simulink model "MATE_9LevelDrive_LowHarmonicRectifier"  (R2024b)
settings: Solver=FixedStepDiscrete  StartTime=0.0  StopTime=1  FixedStep=Ts  RelTol=1e-3
PostLoadFcn:
  | Ts=25e-6; initDrive9Level;Rsnu=30; Csnu=3e-6;Ron=0.01;Roff=1e6; Vf=2;
InitFcn:
  | Ts=25e-6; initDrive9Level;Rsnu=30; Csnu=3e-6;Ron=0.01;Roff=1e6; Vf=2;
values from neighbouring files (symbols this model uses):
  Lbase = Zbase/wbase    (= 0.0044902914611)    [initDrive9Level.m]
  Rgnd_rectifier = 1e4    (= 10000)    [initDrive9Level.m]
  T_2wind_ratio = 0.2677    [initDrive9Level.m]
  T_Lpu = Ltot_pu*9/10    (= 0.036)    [initDrive9Level.m]
  T_Lpu_pri = Ltot_pu/10    (= 0.004)    [initDrive9Level.m]
  T_Rpu = Rtot_pu*9/10    (= 0.009)    [initDrive9Level.m]
  T_Rpu_pri = Rtot_pu/10    (= 0.001)    [initDrive9Level.m]
  T_Vpri = 3000    [initDrive9Level.m]
  T_Vpri_15comp = 1.1168    [initDrive9Level.m]
  T_Vsec = 920    [initDrive9Level.m]
  Zbase = T_Vsec*T_Vsec/T_Pbase    (= 1.6928)    [initDrive9Level.m]
undefined symbols (not defined in the file or in its folder): DiscIntNeverNeededParam, gcbh, sps_rtmsupport
libraries: fl_lib x192, ee_lib x105, simetranss x26, nesl_utility x21
(part 1 of 5)
Description:
  | OHV Parallel Inverter Real-Time Simulator
settings Model: ARTEMISmethode_block_infos=$$__separator__$$  Creator=Kyle
settings SolverCC: AlgebraicLoopSolver=TrustRegion
settings DataIOCC: InitialState=xFinal  LimitDataPoints=on  MaxDataPoints=5000  SaveFormat=StructureWithTime  SignalLoggingSaveFormat=ModelDataLogs  SaveOutput=off  SaveTime=off  ReturnWorkspaceOutputs=off  SignalLoggingName=sigsOut
settings OptimizationCC: BlockReduction=off  BooleanDataType=off  OptimizeBlockIOStorage=off  BufferReuse=off  GlobalBufferReuse=off  ExpressionFolding=off  ExpressionDepthLimit=2147483647  LocalBlockOutputs=off  InitFltsAndDblsToZero=on  LifeSpan=inf
settings DebuggingCC: SaveWithParameterizedLinksMsg=none  UnderspecifiedInitializationDetection=Classic  MergeDetectMultiDrivingBlocksExec=none  SignalResolutionControl=TryResolveAllWithWarning  MultiTaskDSMMsg=warning  MultiTaskCondExecSysMsg=none  FcnCallInpInsideContextMsg=warning  UnconnectedInputMsg=warning  UnconnectedOutputMsg=warning  UnconnectedLineMsg=warning  AllowSymbolicDim=off  StateNameClashWarn=warning  SFUnexpectedBacktrackingDiag=warning  SFNoUnconditionalDefaultTransitionDiag=warning  SFExecutionAtInitializationDiag=none  ArithmeticOperatorsInVariantConditions=warning
settings HardwareCC: ProdBitPerPointer=32  ProdBitPerSizeT=32  ProdBitPerPtrDiffT=32  ProdLargestAtomicFloat=None  ProdIntDivRoundTo=Undefined  ProdEndianess=Unspecified  ProdWordSize=32  ProdHWDeviceType=32-bit Generic  TargetUnknown=on
settings ModelReferenceCC: EnableRefExpFcnMdlSchedulingChecks=on  PropagateSignalLabelsOutOfModel=off
settings SFSimCC: SimUseLocalCustomCode=off  CustomCodeUndefinedFunction=UseInterfaceOnly
settings RTWCC: RTWUseLocalCustomCode=off  GPUComputeCapability=3.5
settings CodeAppCC: StateflowObjectComments=on
settings GRTTargetCC: TargetFcnLib=ansi_tfl_tmw.mat  TargetLangStandard=C89/C90 (ANSI)  CombineOutputUpdateFcns=off  GRTInterface=on
settings ConfigComp: CovMetricSettings=dw  CovSaveCumulativeToWorkspaceVar=on  CovSaveSingleToWorkspaceVar=on  CovExternalEMLEnable=off
settings SimscapeCC: SimscapeNormalizeSystem=off

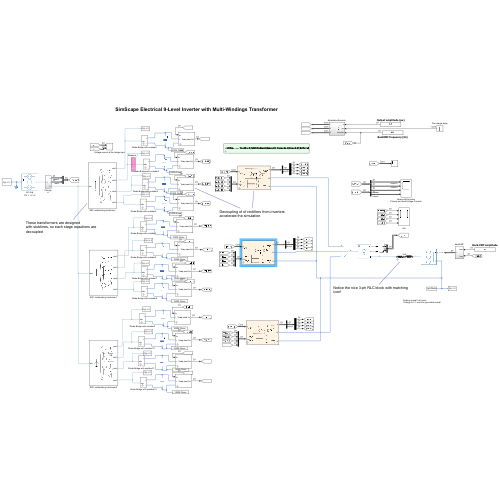
[thumbnail: Simulink's stored preview of the top-level diagram]
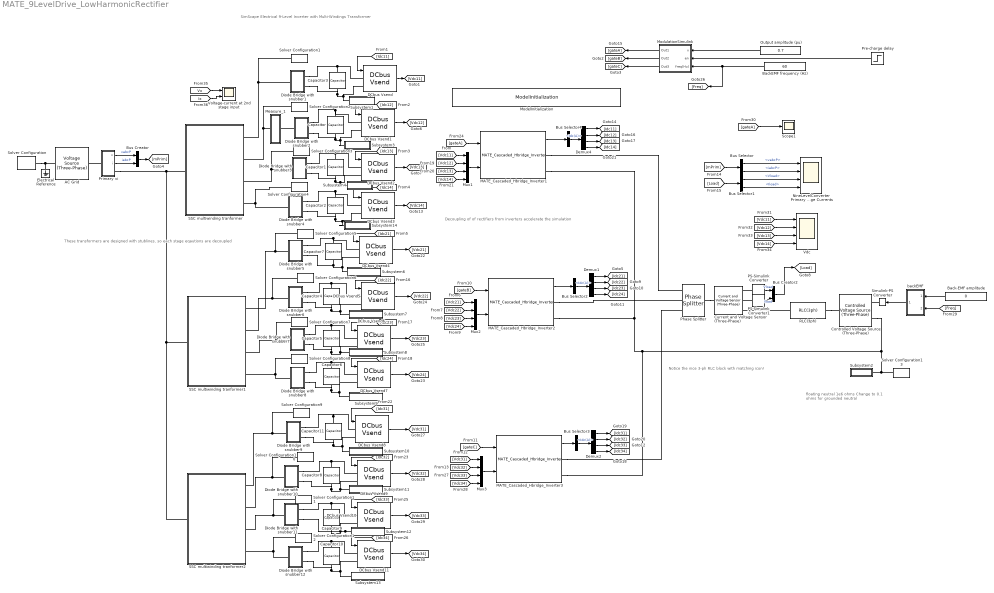
== system MATE_9LevelDrive_LowHarmonicRectifier ==
  note: Decoupling of of rectifiers from inverters
      | accelerate the simulation
  note: floating neutral 1e6 ohms
      | Change to 0.1 ohms for grounded neutral
  note: SimScape Electrical 9-Level Inverter with Multi-Windings Transformer
  note: These transformers are designed
      | with stublines, so each stage eqautions are decoupled
  note: Notice the nice 3-ph RLC block with matching icon!
  AC Grid : ee_lib/Sources/Voltage Source (Three-Phase)  vline_rms=120*sqrt(3) V  shift=0 deg  freq=60 Hz  impedance_option=1  SShortCircuit=1e6 A*V  XR=15  R=0.01 Ohm  L=3.97e-4 H  harmonic_option=0  harmonic_orders=[5.0, 7.0, 11.0, 13.0]  harmonic_ratios=[0.1, 0.1, 0.1, 0.1]  G_parasitic=0 1/Ohm  I_specify=off  I_priority=None  I=[0, 0, 0] A  I_nominal_specify=off  I_nominal_value=1  I_nominal_unit=A
      settings: AttributesFormatString="208 V  60 Hz"
  Back-EMF amplitude : Constant  Value=0
  BackEMF frequency (Hz) : Constant  Value=60
  Bus Creator : BusCreator  Inputs=2
  Bus Creator2 : BusCreator  Inputs=2
  Bus Selector : BusSelector  OutputSignals=vabcP,iabcP
  Bus Selector1 : BusSelector  OutputSignals=Vload,Iload
  Bus Selector2 : BusSelector  OutputSignals=Idc(A)
  Bus Selector3 : BusSelector  OutputSignals=Idc(A)
  Bus Selector4 : BusSelector  OutputSignals=Idc(A)
  Capacitor{,1..11} (12 alike) : fl_lib/Electrical/Electrical Elements/Capacitor  c=Cdclink F  r=Rdclink_series Ohm  g=0 1/Ohm  i_specify=off  i_priority=None  i=0 A  i_nominal_specify=off  i_nominal_value=1  i_nominal_unit=A  v_specify=off  v_priority=None  v=0 V  v_nominal_specify=off  v_nominal_value=1  v_nominal_unit=V  vc_specify=off  vc_priority=High  vc=0 V  vc_nominal_specify=off  vc_nominal_value=1  vc_nominal_unit=V
  Controlled Voltage Source (Three-Phase) : ee_lib/Sources/Controlled Voltage Source (Three-Phase)  input_option=ee.enum.inputType.instantaneous  FRated=60 Hz
      settings: InternalSimscapePortConfiguration="{\"Bottom\":[],\"Left\":[{\"id\":\"S\",\"label\":\"S\",\"type\":\"input\"},{\"id\":\"n\",\"label\":\"n\",\"type\":\"foundation.electrical.electrical\"}],\"Right\":[{\"id\":\"N\",\"label\":\"~\",\"type\":\"foundation.electrical.three_phase\"}],\"Top\":[]}"
  Current and Voltage Sensor (Three-Phase) : ee_lib/Sensors & Transducers/Current and Voltage Sensor (Three-Phase)  vMeasurementType=ee.enum.vmeasurement.lg  outputUnit=ee.enum.unit.si  SRated=100e6 A*V  VRated=24e3 V  I_specify=off  I_priority=None  I=[0, 0, 0] A  I_nominal_specify=off  I_nominal_value=1  I_nominal_unit=A  V_specify=off  V_priority=None  V=[0, 0, 0] V  V_nominal_specify=off  V_nominal_value=1  V_nominal_unit=V
      settings: InternalSimscapePortConfiguration="{\"Bottom\":[],\"Left\":[{\"id\":\"N1\",\"label\":\"~1\",\"type\":\"foundation.electrical.three_phase\"}],\"Right\":[{\"id\":\"V_output\",\"label\":\"V\",\"type\":\"output\"},{\"id\":\"I_output\",\"label\":\"I\",\"type\":\"output\"},{\"id\":\"N2\",\"label\":\"~2\",\"type\":\"foundation.electrical.three_phase\"}],\"Top\":[]}"
  DCbus Vsend{,1..11} (12 alike) : simetranss/Network decoupling/DCbus Vsend  Ts=Ts
  Demux1 : Demux
      settings: DisplayOption=none
  Demux2 : Demux
      settings: DisplayOption=none
  Demux4 : Demux
      settings: DisplayOption=none
  Diode Bridge with snubber1 : Subsystem  mask(MATE 3-phase Diode/Thyristor Rectifier){rsnu=Rsnu, csnu=Csnu}
      mask prompts: rsnu "Snubber resistance (Ohms)"; csnu "Snubber capacitance (Ohms)"
  Diode Bridge with snubber10 : Subsystem  mask(MATE 3-phase Diode/Thyristor Rectifier){rsnu=Rsnu, csnu=Csnu}
      mask prompts: rsnu "Snubber resistance (Ohms)"; csnu "Snubber capacitance (Ohms)"
  Diode Bridge with snubber11 : Subsystem  mask(MATE 3-phase Diode/Thyristor Rectifier){rsnu=Rsnu, csnu=Csnu}
      mask prompts: rsnu "Snubber resistance (Ohms)"; csnu "Snubber capacitance (Ohms)"
  Diode Bridge with snubber12 : Subsystem  mask(MATE 3-phase Diode/Thyristor Rectifier){rsnu=Rsnu, csnu=Csnu}
      mask prompts: rsnu "Snubber resistance (Ohms)"; csnu "Snubber capacitance (Ohms)"
  Diode Bridge with snubber2 : Subsystem  mask(MATE 3-phase Diode/Thyristor Rectifier){rsnu=Rsnu, csnu=Csnu}
      mask prompts: rsnu "Snubber resistance (Ohms)"; csnu "Snubber capacitance (Ohms)"
  Diode Bridge with snubber3 : Subsystem  mask(MATE 3-phase Diode/Thyristor Rectifier){rsnu=Rsnu, csnu=Csnu}
      mask prompts: rsnu "Snubber resistance (Ohms)"; csnu "Snubber capacitance (Ohms)"
  Diode Bridge with snubber4 : Subsystem  mask(MATE 3-phase Diode/Thyristor Rectifier){rsnu=Rsnu, csnu=Csnu}
      mask prompts: rsnu "Snubber resistance (Ohms)"; csnu "Snubber capacitance (Ohms)"
  Diode Bridge with snubber5 : Subsystem  mask(MATE 3-phase Diode/Thyristor Rectifier){rsnu=Rsnu, csnu=Csnu}
      mask prompts: rsnu "Snubber resistance (Ohms)"; csnu "Snubber capacitance (Ohms)"
  Diode Bridge with snubber6 : Subsystem  mask(MATE 3-phase Diode/Thyristor Rectifier){rsnu=Rsnu, csnu=Csnu}
      mask prompts: rsnu "Snubber resistance (Ohms)"; csnu "Snubber capacitance (Ohms)"
  Diode Bridge with snubber7 : Subsystem  mask(MATE 3-phase Diode/Thyristor Rectifier){rsnu=Rsnu, csnu=Csnu}
      mask prompts: rsnu "Snubber resistance (Ohms)"; csnu "Snubber capacitance (Ohms)"
  Diode Bridge with snubber8 : Subsystem  mask(MATE 3-phase Diode/Thyristor Rectifier){rsnu=Rsnu, csnu=Csnu}
      mask prompts: rsnu "Snubber resistance (Ohms)"; csnu "Snubber capacitance (Ohms)"
  Diode Bridge with snubber9 : Subsystem  mask(MATE 3-phase Diode/Thyristor Rectifier){rsnu=Rsnu, csnu=Csnu}
      mask prompts: rsnu "Snubber resistance (Ohms)"; csnu "Snubber capacitance (Ohms)"
  Electrical Reference : fl_lib/Electrical/Electrical Elements/Electrical Reference
  MATE_Cascaded_Hbridge_Inverter1 : simetranss/Power converters/MATE_Cascaded_Hbridge_Inverter  Gtype=Mean Active Duty (0<=g<=1)  nbc=4  ron=0.001  roff=1e5  Ts=Ts
  MATE_Cascaded_Hbridge_Inverter2 : simetranss/Power converters/MATE_Cascaded_Hbridge_Inverter  Gtype=Mean Active Duty (0<=g<=1)  nbc=4  ron=0.001  roff=1e5  Ts=Ts
  MATE_Cascaded_Hbridge_Inverter3 : simetranss/Power converters/MATE_Cascaded_Hbridge_Inverter  Gtype=Mean Active Duty (0<=g<=1)  nbc=4  ron=0.001  roff=1e5  Ts=Ts
  Measure_1 : Subsystem  DialogController=POWERSYS.PowerSysDialog  StartFcn=sps_rtmsupport('StartFcn',gcbh);  StopFcn=sps_rtmsupport('StopFcn',gcbh);  mask(Three-Phase Measurement){Va=Vx, Ia=Ix}
      mask prompts: Va "Voltage signal label  (use a From block to collect this signal)"; Ia "Current signal label  (use a From block to collect this signal)"
      mask help:
      | Ideal three-phase voltage and current measurements.
      |
      | The block outputs the voltages and currents in volts and amperes at the corresponding From blocks
      mask init:
      | bloc = gcb;
      | 
      | Vtag=get_param(bloc,'Va');
      | Itag=get_param(bloc,'Ia');
      | 
      | set_param([bloc '/Vabc'],'GotoTag',[Vtag]);
      | set_param([bloc '/Iabc'],'GotoTag',[Itag]);
      settings: UndoDeleteFcn=sps_rtmsupport('UndoDeleteFcn',gcbh);
      mask Help: helpview(psbhelp)
  ModelInitialization : simetranss/Usefulls/ModelInitialization  InitFcnX=Ts=25e-6; initDrive9Level;Rsnu=30; Csnu=3e-6;Ron=0.01;Roff=1e6; Vf=2;  prel=off  posl=on  inif=on  strf=off
  ModulationSimulink : Subsystem
  Mux1 : Mux
  Mux2 : Mux
  Mux3 : Mux
  NineLevelConverter Primary and load Voltage Currents : Scope  NumInputPorts=4
  Output amplitude (pu) : Constant  Value=0.7
  PS-Simulink Converter : nesl_utility/PS-Simulink Converter  PhysicalDomain=network_engine_domain  SubClassName=ps_output  LeftPortType=input  RightPortType=output  PseudoPeriodic=off  Frequencies=[]  VectorFormat=1-D array  Unit=V  AffineConversion=off
  PS-Simulink Converter1 : nesl_utility/PS-Simulink Converter  PhysicalDomain=network_engine_domain  SubClassName=ps_output  LeftPortType=input  RightPortType=output  PseudoPeriodic=off  Frequencies=[]  VectorFormat=1-D array  Unit=A  AffineConversion=off
  Phase Splitter : ee_lib/Connectors & References/Phase Splitter
  Pre-charge delay : Step  Time=0.2  SampleTime=0
  Primary vi : Subsystem
  RLC(3ph) : simetranss/Passive/RLC(3ph)  BranchType=RL  SerPar=Series  Resistance=5  Inductance=6e-3  Capacitance=1e-6  Ropen=1e9
  SSC multiwinding tranformer : Subsystem
  SSC multiwinding tranformer1 : Subsystem
  SSC multiwinding tranformer2 : Subsystem
  Scope1 : Scope
  Simulink-PS Converter : nesl_utility/Simulink-PS Converter  PhysicalDomain=network_engine_domain  SubClassName=ps_input  LeftPortType=input  RightPortType=output  PseudoPeriodic=off  Frequencies=[]  NoiseDistribution=none  NoiseParameters=[]  Unit=1  AffineConversion=off  FilteringAndDerivatives=provide  SimscapeFilterOrder=1  InputFilterTimeConstant=0.001  UdotUserProvided=0
  Solver Configuration : nesl_utility/Solver Configuration  PhysicalDomain=network_engine_domain  SubClassName=solver  LeftPortType=input  RightPortType=generic  Tones=[]  Harmonics=[]  SimulateNoise=off  Profile=off  UseLocalSampling=off  EnableSwitchedLinearOptims=on  FrequencyDomain=off  UseCCode=off  RelTol=0.001  AbsTol=1e-06  MinStep=1e-09  ToWorkspace=off  RevertToSquareIcSolve=off  NumHomotopyIterations=100  PhasorMode=off  PhasorModeNumHarmonics=1  ConsistencySolver=NEWTON_FTOL  IndexReductionMethod=None  DoDC=off  ResidualTolerance=1e-03  ConsistencyTolSource=GLOBAL  ConsistencyAbsTol=0.001  ConsistencyRelTol=0.001  ConsistencyTolFactor=0.001  UseLocalSolver=on  LocalSolverChoice=NE_BACKWARD_EULER_ADVANCER  ResolveIndetEquations=off  FunctionEvalNumThread=1  LocalSolverSampleTime=Ts  DoFixedCost=on  MaxNonlinIter=1  MaxModeIter=2  ComputeImpulses=off  ImpulseIterations=2  LinearAlgebra=auto  LinearAlgebraNumThread=0  EquationFormulation=NE_TIME_EF  DelaysMemoryBudget=1024  AutomaticFiltering=off  FilteringTimeConstant=0.001  PartitionStorageMethod=AS_NEEDED  PartitionMemoryBudget=1024  PartitionMethod=ROBUST  MultibodyUseLocalSolver=off  MultibodyLocalSolverChoice=ODE1  MultibodyLocalSolverSampleTime=0.001
  Solver Configuration{1..12} (12 alike) : nesl_utility/Solver Configuration  PhysicalDomain=network_engine_domain  SubClassName=solver  LeftPortType=input  RightPortType=generic  Tones=[]  Harmonics=[]  SimulateNoise=off  Profile=off  UseLocalSampling=off  EnableSwitchedLinearOptims=on  FrequencyDomain=off  UseCCode=off  RelTol=0.001  AbsTol=1e-06  MinStep=1e-09  ToWorkspace=off  RevertToSquareIcSolve=off  NumHomotopyIterations=100  PhasorMode=off  PhasorModeNumHarmonics=1  ConsistencySolver=NEWTON_FTOL  IndexReductionMethod=None  DoDC=off  ResidualTolerance=1e-09  ConsistencyTolSource=GLOBAL  ConsistencyAbsTol=0.001  ConsistencyRelTol=0.001  ConsistencyTolFactor=0.001  UseLocalSolver=on  LocalSolverChoice=NE_BACKWARD_EULER_ADVANCER  ResolveIndetEquations=off  FunctionEvalNumThread=1  LocalSolverSampleTime=Ts  DoFixedCost=on  MaxNonlinIter=1  MaxModeIter=2  ComputeImpulses=off  ImpulseIterations=2  LinearAlgebra=auto  LinearAlgebraNumThread=0  EquationFormulation=NE_TIME_EF  DelaysMemoryBudget=1024  AutomaticFiltering=off  FilteringTimeConstant=0.001  PartitionStorageMethod=AS_NEEDED  PartitionMemoryBudget=1024  PartitionMethod=ROBUST  MultibodyUseLocalSolver=off  MultibodyLocalSolverChoice=ODE1  MultibodyLocalSolverSampleTime=0.001
  Solver Configuration13 : nesl_utility/Solver Configuration  PhysicalDomain=network_engine_domain  SubClassName=solver  LeftPortType=input  RightPortType=generic  Tones=[]  Harmonics=[]  SimulateNoise=off  Profile=off  UseLocalSampling=off  EnableSwitchedLinearOptims=on  FrequencyDomain=off  UseCCode=off  RelTol=0.001  AbsTol=1e-06  MinStep=1e-09  ToWorkspace=off  RevertToSquareIcSolve=off  NumHomotopyIterations=100  PhasorMode=off  PhasorModeNumHarmonics=1  ConsistencySolver=NEWTON_FTOL  IndexReductionMethod=None  DoDC=off  ResidualTolerance=1e-03  ConsistencyTolSource=GLOBAL  ConsistencyAbsTol=0.001  ConsistencyRelTol=0.001  ConsistencyTolFactor=0.001  UseLocalSolver=on  LocalSolverChoice=NE_BACKWARD_EULER_ADVANCER  ResolveIndetEquations=off  FunctionEvalNumThread=1  LocalSolverSampleTime=Ts  DoFixedCost=on  MaxNonlinIter=1  MaxModeIter=2  ComputeImpulses=off  ImpulseIterations=2  LinearAlgebra=auto  LinearAlgebraNumThread=0  EquationFormulation=NE_TIME_EF  DelaysMemoryBudget=1024  AutomaticFiltering=off  FilteringTimeConstant=0.001  PartitionStorageMethod=AS_NEEDED  PartitionMemoryBudget=1024  PartitionMethod=ROBUST  MultibodyUseLocalSolver=off  MultibodyLocalSolverChoice=ODE1  MultibodyLocalSolverSampleTime=0.001
  Subsystem1 : Subsystem  mask(Ground Referencing Resistor){Rr=Rgnd_rectifier}
      mask prompts: Rr "Resistance (Ohms)"
      mask help: This block is a simple resistance to provide a reference to the ground for the SimScape solver.
      mask init:
      | r=get_param(gcb,'Rr');
      | rr=num2str(Rr);
      | txt=[rr ' Ohms'];
      mask Display: disp(txt)
  Subsystem10 : Subsystem  mask(Ground Referencing Resistor){Rr=Rgnd_rectifier}
      mask prompts: Rr "Resistance (Ohms)"
      mask help: This block is a simple resistance to provide a reference to the ground for the SimScape solver.
      mask init:
      | r=get_param(gcb,'Rr');
      | rr=num2str(Rr);
      | txt=[rr ' Ohms'];
      mask Display: disp(txt)
  Subsystem11 : Subsystem  mask(Ground Referencing Resistor){Rr=Rgnd_rectifier}
      mask prompts: Rr "Resistance (Ohms)"
      mask help: This block is a simple resistance to provide a reference to the ground for the SimScape solver.
      mask init:
      | r=get_param(gcb,'Rr');
      | rr=num2str(Rr);
      | txt=[rr ' Ohms'];
      mask Display: disp(txt)
  Subsystem12 : Subsystem  mask(Ground Referencing Resistor){Rr=Rgnd_rectifier}
      mask prompts: Rr "Resistance (Ohms)"
      mask help: This block is a simple resistance to provide a reference to the ground for the SimScape solver.
      mask init:
      | r=get_param(gcb,'Rr');
      | rr=num2str(Rr);
      | txt=[rr ' Ohms'];
      mask Display: disp(txt)
  Subsystem13 : Subsystem  mask(Ground Referencing Resistor){Rr=Rgnd_rectifier}
      mask prompts: Rr "Resistance (Ohms)"
      mask help: This block is a simple resistance to provide a reference to the ground for the SimScape solver.
      mask init:
      | r=get_param(gcb,'Rr');
      | rr=num2str(Rr);
      | txt=[rr ' Ohms'];
      mask Display: disp(txt)
  Subsystem14 : Subsystem  mask(Ground Referencing Resistor){Rr=Rgnd_rectifier}
      mask prompts: Rr "Resistance (Ohms)"
      mask help: This block is a simple resistance to provide a reference to the ground for the SimScape solver.
      mask init:
      | r=get_param(gcb,'Rr');
      | rr=num2str(Rr);
      | txt=[rr ' Ohms'];
      mask Display: disp(txt)
  Subsystem2 : Subsystem  mask(Ground Referencing Resistor){Rr=1e6}
      mask prompts: Rr "Resistance (Ohms)"
      mask help: This block is a simple resistance to provide a reference to the ground for the SimScape solver.
      mask init:
      | r=get_param(gcb,'Rr');
      | txt=[r ' Ohms'];
      mask Display: disp(txt)
  Subsystem3 : Subsystem  mask(Ground Referencing Resistor){Rr=Rgnd_rectifier}
      mask prompts: Rr "Resistance (Ohms)"
      mask help: This block is a simple resistance to provide a reference to the ground for the SimScape solver.
      mask init:
      | r=get_param(gcb,'Rr');
      | rr=num2str(Rr);
      | txt=[rr ' Ohms'];
      mask Display: disp(txt)
  Subsystem4 : Subsystem  mask(Ground Referencing Resistor){Rr=Rgnd_rectifier}
      mask prompts: Rr "Resistance (Ohms)"
      mask help: This block is a simple resistance to provide a reference to the ground for the SimScape solver.
      mask init:
      | r=get_param(gcb,'Rr');
      | rr=num2str(Rr);
      | txt=[rr ' Ohms'];
      mask Display: disp(txt)
  Subsystem6 : Subsystem  mask(Ground Referencing Resistor){Rr=Rgnd_rectifier}
      mask prompts: Rr "Resistance (Ohms)"
      mask help: This block is a simple resistance to provide a reference to the ground for the SimScape solver.
      mask init:
      | r=get_param(gcb,'Rr');
      | rr=num2str(Rr);
      | txt=[rr ' Ohms'];
      mask Display: disp(txt)
  Subsystem7 : Subsystem  mask(Ground Referencing Resistor){Rr=Rgnd_rectifier}
      mask prompts: Rr "Resistance (Ohms)"
      mask help: This block is a simple resistance to provide a reference to the ground for the SimScape solver.
      mask init:
      | r=get_param(gcb,'Rr');
      | rr=num2str(Rr);
      | txt=[rr ' Ohms'];
      mask Display: disp(txt)
  Subsystem8 : Subsystem  mask(Ground Referencing Resistor){Rr=Rgnd_rectifier}
      mask prompts: Rr "Resistance (Ohms)"
      mask help: This block is a simple resistance to provide a reference to the ground for the SimScape solver.
      mask init:
      | r=get_param(gcb,'Rr');
      | rr=num2str(Rr);
      | txt=[rr ' Ohms'];
      mask Display: disp(txt)
  Subsystem9 : Subsystem  mask(Ground Referencing Resistor){Rr=Rgnd_rectifier}
      mask prompts: Rr "Resistance (Ohms)"
      mask help: This block is a simple resistance to provide a reference to the ground for the SimScape solver.
      mask init:
      | r=get_param(gcb,'Rr');
      | rr=num2str(Rr);
      | txt=[rr ' Ohms'];
      mask Display: disp(txt)
  Vdc : Scope  NumInputPorts=4
  Voltage-current at 2nd stage input : Scope  NumInputPorts=2
  backEMF : Subsystem
  wires:
  Bus Creator/1 -> [mPrim]
  Primary vi/1(v) -> Bus Creator/1  "vabcP"
  Primary vi/2(i) -> Bus Creator/2  "iabcP"
  DCbus Vsend1/1 -> [Vdc12]
  DCbus Vsend2/1 -> [Vdc13]
  DCbus Vsend3/1 -> [Vdc14]
  DCbus Vsend/1 -> [Vdc11]
  Back-EMF amplitude/1 -> backEMF/1(amp)
  backEMF/1(Out1) -> Simulink-PS Converter/1
  BackEMF frequency (Hz)/1 -> [Freq], ModulationSimulink/3(freq(Hz))
  Output amplitude (pu)/1 -> ModulationSimulink/1(x)
  [mPrim] -> Bus Selector/1
  PS-Simulink Converter1/1 -> Bus Creator2/2  "Iload"
  PS-Simulink Converter/1 -> Bus Creator2/1  "Vload"
  Bus Creator2/1 -> [Load]
  [Load] -> Bus Selector1/1
  Bus Selector/2 -> NineLevelConverter Primary and load Voltage Currents/2  "<iabcP>"
  Bus Selector/1 -> NineLevelConverter Primary and load Voltage Currents/1  "<vabcP>"
  Bus Selector1/2 -> NineLevelConverter Primary and load Voltage Currents/4  "<Iload>"
  Bus Selector1/1 -> NineLevelConverter Primary and load Voltage Currents/3  "<Vload>"
  ModulationSimulink/1(Out1) -> [gateA]
  [Vdc11] -> Mux1/1
  [Vdc12] -> Mux1/2
  [Vdc13] -> Mux1/3
  [Vdc14] -> Mux1/4
  Mux1/1 -> MATE_Cascaded_Hbridge_Inverter1/2
  [gateA] -> MATE_Cascaded_Hbridge_Inverter1/1
  MATE_Cascaded_Hbridge_Inverter1/1 -> Bus Selector4/1
  Bus Selector4/1 -> Demux4/1  "<Idc(A)>"
  Demux4/1 -> [Idc11]
  Demux4/2 -> [Idc12]
  Demux4/3 -> [Idc13]
  Demux4/4 -> [Idc14]
  [Idc11] -> DCbus Vsend/1
  [Idc12] -> DCbus Vsend1/1
  [Idc13] -> DCbus Vsend2/1
  [Idc14] -> DCbus Vsend3/1
  Pre-charge delay/1 -> ModulationSimulink/2(en)
  DCbus Vsend4/1 -> [Vdc21]
  DCbus Vsend5/1 -> [Vdc22]
  DCbus Vsend6/1 -> [Vdc23]
  DCbus Vsend7/1 -> [Vdc24]
  [Idc21] -> DCbus Vsend4/1
  [Idc22] -> DCbus Vsend5/1
  [Idc23] -> DCbus Vsend6/1
  [Idc24] -> DCbus Vsend7/1
  DCbus Vsend8/1 -> [Vdc31]
  DCbus Vsend9/1 -> [Vdc32]
  DCbus Vsend10/1 -> [Vdc33]
  DCbus Vsend11/1 -> [Vdc34]
  [Idc31] -> DCbus Vsend8/1
  [Idc32] -> DCbus Vsend9/1
  [Idc33] -> DCbus Vsend10/1
  [Idc34] -> DCbus Vsend11/1
  ModulationSimulink/2(Out2) -> [gateB]
  ModulationSimulink/3(Out3) -> [gateC]
  Demux1/4 -> [Idc24]
  Demux1/3 -> [Idc23]
  Demux1/2 -> [Idc22]
  Demux1/1 -> [Idc21]
  Bus Selector2/1 -> Demux1/1  "<Idc(A)>"
  MATE_Cascaded_Hbridge_Inverter2/1 -> Bus Selector2/1
  [gateB] -> MATE_Cascaded_Hbridge_Inverter2/1
  Mux2/1 -> MATE_Cascaded_Hbridge_Inverter2/2
  [Vdc24] -> Mux2/4
  [Vdc23] -> Mux2/3
  [Vdc22] -> Mux2/2
  [Vdc21] -> Mux2/1
  [Vdc31] -> Mux3/1
  [Vdc32] -> Mux3/2
  [Vdc33] -> Mux3/3
  [Vdc34] -> Mux3/4
  Mux3/1 -> MATE_Cascaded_Hbridge_Inverter3/2
  [gateC] -> MATE_Cascaded_Hbridge_Inverter3/1
  MATE_Cascaded_Hbridge_Inverter3/1 -> Bus Selector3/1
  Bus Selector3/1 -> Demux2/1  "<Idc(A)>"
  Demux2/1 -> [Idc31]
  Demux2/2 -> [Idc32]
  Demux2/3 -> [Idc33]
  Demux2/4 -> [Idc34]
  [Freq] -> backEMF/2(freq)
  [gateA] -> Scope1/1
  [Vdc11] -> Vdc/1
  [Vdc12] -> Vdc/2
  [Vdc13] -> Vdc/3
  [Vdc14] -> Vdc/4
  [Vx] -> Voltage-current at 2nd stage input/1
  [Ix] -> Voltage-current at 2nd stage input/2
  connections:
  AC Grid/LConn1 -- Solver Configuration/RConn1 -- Electrical Reference/LConn1
  Primary vi/RConn1 -- SSC multiwinding tranformer/LConn1 -- SSC multiwinding tranformer2/LConn1 -- SSC multiwinding tranformer1/LConn1
  Primary vi/LConn1 -- AC Grid/RConn1
  Capacitor/LConn1 -- Diode Bridge with snubber2/RConn1 -- DCbus Vsend1/LConn1
  Capacitor/RConn1 -- Diode Bridge with snubber2/RConn2 -- DCbus Vsend1/LConn2 -- Subsystem3/RConn1
  Diode Bridge with snubber3/RConn1 -- DCbus Vsend2/LConn1 -- Capacitor1/LConn1
  Capacitor1/RConn1 -- Diode Bridge with snubber3/RConn2 -- DCbus Vsend2/LConn2 -- Subsystem4/RConn1
  Capacitor2/LConn1 -- DCbus Vsend3/LConn1 -- Diode Bridge with snubber4/RConn1
  Capacitor2/RConn1 -- Diode Bridge with snubber4/RConn2 -- DCbus Vsend3/LConn2 -- Subsystem14/RConn1
  Capacitor3/LConn1 -- DCbus Vsend/LConn1 -- Diode Bridge with snubber1/RConn1
  Capacitor3/RConn1 -- Diode Bridge with snubber1/RConn2 -- DCbus Vsend/LConn2 -- Subsystem1/RConn1
  Diode Bridge with snubber1/LConn1 -- SSC multiwinding tranformer/RConn1 -- Solver Configuration1/RConn1
  Measure_1/LConn1 -- Solver Configuration2/RConn1 -- SSC multiwinding tranformer/RConn2
  Diode Bridge with snubber3/LConn1 -- SSC multiwinding tranformer/RConn3 -- Solver Configuration3/RConn1
  Diode Bridge with snubber4/LConn1 -- Solver Configuration4/RConn1 -- SSC multiwinding tranformer/RConn4
  RLC(3ph)/RConn1 -- Controlled Voltage Source (Three-Phase)/RConn1
  Simulink-PS Converter/RConn1 -- Controlled Voltage Source (Three-Phase)/LConn1
  Phase Splitter/LConn1 -- Current and Voltage Sensor (Three-Phase)/LConn1
  RLC(3ph)/LConn1 -- Current and Voltage Sensor (Three-Phase)/RConn3
  PS-Simulink Converter/LConn1 -- Current and Voltage Sensor (Three-Phase)/RConn1
  PS-Simulink Converter1/LConn1 -- Current and Voltage Sensor (Three-Phase)/RConn2
  Controlled Voltage Source (Three-Phase)/LConn2 -- Solver Configuration13/RConn1 -- Subsystem2/RConn1 -- MATE_Cascaded_Hbridge_Inverter3/RConn2 -- MATE_Cascaded_Hbridge_Inverter2/RConn2 -- MATE_Cascaded_Hbridge_Inverter1/RConn2
  Diode Bridge with snubber6/RConn1 -- DCbus Vsend5/LConn1 -- Capacitor4/LConn1
  Capacitor4/RConn1 -- Diode Bridge with snubber6/RConn2 -- DCbus Vsend5/LConn2 -- Subsystem7/RConn1
  Diode Bridge with snubber7/RConn1 -- DCbus Vsend6/LConn1 -- Capacitor5/LConn1
  Capacitor5/RConn1 -- Diode Bridge with snubber7/RConn2 -- DCbus Vsend6/LConn2 -- Subsystem8/RConn1
  Capacitor6/LConn1 -- DCbus Vsend7/LConn1 -- Diode Bridge with snubber8/RConn1
  Capacitor6/RConn1 -- Diode Bridge with snubber8/RConn2 -- DCbus Vsend7/LConn2 -- Subsystem9/RConn1
  Diode Bridge with snubber5/RConn1 -- DCbus Vsend4/LConn1 -- Capacitor7/LConn1
  Capacitor7/RConn1 -- Diode Bridge with snubber5/RConn2 -- DCbus Vsend4/LConn2 -- Subsystem6/RConn1
  Diode Bridge with snubber8/LConn1 -- Solver Configuration8/RConn1 -- SSC multiwinding tranformer1/RConn4
  Diode Bridge with snubber7/LConn1 -- SSC multiwinding tranformer1/RConn3 -- Solver Configuration7/RConn1
  Diode Bridge with snubber6/LConn1 -- SSC multiwinding tranformer1/RConn2 -- Solver Configuration6/RConn1
  Diode Bridge with snubber5/LConn1 -- SSC multiwinding tranformer1/RConn1 -- Solver Configuration5/RConn1
  Capacitor8/LConn1 -- DCbus Vsend9/LConn1 -- Diode Bridge with snubber10/RConn1
  Capacitor8/RConn1 -- Diode Bridge with snubber10/RConn2 -- DCbus Vsend9/LConn2 -- Subsystem11/RConn1
  Capacitor9/LConn1 -- DCbus Vsend10/LConn1 -- Diode Bridge with snubber11/RConn1
  Subsystem12/RConn1 -- DCbus Vsend10/LConn2 -- Diode Bridge with snubber11/RConn2 -- Capacitor9/RConn1
  Capacitor10/LConn1 -- DCbus Vsend11/LConn1 -- Diode Bridge with snubber12/RConn1
  Capacitor10/RConn1 -- Diode Bridge with snubber12/RConn2 -- DCbus Vsend11/LConn2 -- Subsystem13/RConn1
  Capacitor11/LConn1 -- DCbus Vsend8/LConn1 -- Diode Bridge with snubber9/RConn1
  Capacitor11/RConn1 -- Diode Bridge with snubber9/RConn2 -- DCbus Vsend8/LConn2 -- Subsystem10/RConn1
  Diode Bridge with snubber9/LConn1 -- SSC multiwinding tranformer2/RConn1 -- Solver Configuration9/RConn1
  Diode Bridge with snubber10/LConn1 -- SSC multiwinding tranformer2/RConn2 -- Solver Configuration10/RConn1
  Diode Bridge with snubber11/LConn1 -- Solver Configuration11/RConn1 -- SSC multiwinding tranformer2/RConn3
  Diode Bridge with snubber12/LConn1 -- Solver Configuration12/RConn1 -- SSC multiwinding tranformer2/RConn4
  MATE_Cascaded_Hbridge_Inverter1/RConn1 -- Phase Splitter/RConn1
  MATE_Cascaded_Hbridge_Inverter2/RConn1 -- Phase Splitter/RConn2
  MATE_Cascaded_Hbridge_Inverter3/RConn1 -- Phase Splitter/RConn3
  Diode Bridge with snubber2/LConn1 -- Measure_1/RConn1

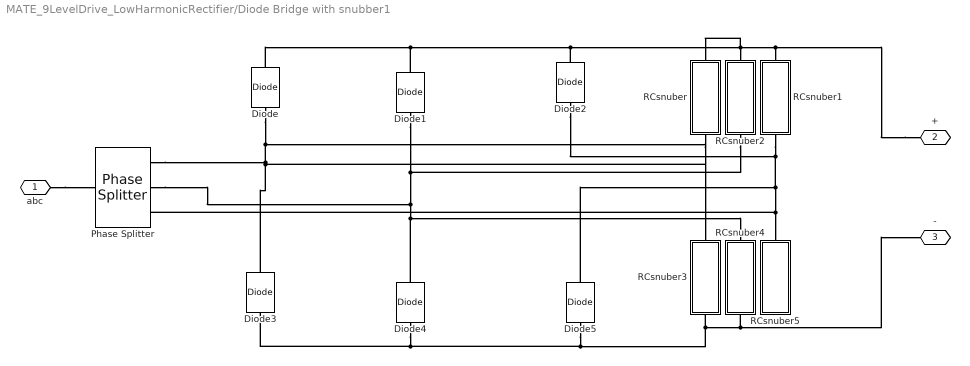
== system MATE_9LevelDrive_LowHarmonicRectifier/Diode Bridge with snubber1 ==
  Diode{,1..5} (6 alike) : ee_lib/Semiconductors & Converters/Diode  ModelType=ee.enum.diode.modelType.pwl  TableType=ee.enum.diode.tableType.IfMat  IfMat=[.07, .12, .19, 1.75, 4.24, 7.32, 11.2; .16, .3, .72, 2.14, 5.02, 8.35, 13.12] A  VfMat=[.9, 1.15, 1.25, 1.5, 1.75, 2.17, 2.6, 2.85; .58, .68, .75, 1.1, 1.38, 1.77, 2.27, 2.7] V  TjVec=[25, 125] degC  VfVec=[.5, .7, .9, 1.3, 1.7, 2.1, 2.5] V  IfVec=[.1, .2, .5, 1, 2, 4, 7, 10] A  IrMat=[1e-06, 2e-06, 5e-06, 1e-05, 2.5e-05, 5e-05, .0001; 2e-06, 5e-06, 1e-05, 4e-05, 8e-05, .0002, .0005] A  VrMat=[10, 100, 200, 250, 300, 325, 350; 10, 70, 160, 220, 270, 300, 320] V  VrVec=[10, 20, 40, 50, 70, 80, 100] V  IrVec=[1e-06, 2e-06, 5e-06, 1e-05, 2e-05, 5e-05, .0001] A  Vf=1 V  Ron=0.01 Ohm  Goff=1e-8 S  prmExp=ee.enum.diode.expParam.useTwo  I12=[.0137, .545] A  V12=[.6, .7] V  RS=0 Ohm  Tmeas=298.15 K  IS=1e-12 A  ec=1  I1=0.0137 A  V1=0.6 V  N_series=1  N_parallel=1  ZenerEnable=false  Rz=0.3 Ohm  BV=inf V  C_param=ee.enum.diode.capParam.fixed  CJ=0 pF  CJ0=5 pF  Vvec=[.1, 10, 100] V  Cvec=[3.5, 1, .4] pF  VJ=1 V  Mgrad=0.5  FC=0.5  Q_param=ee.enum.diode.recoveryParam.off  iRM=-7.15 A  iF=4 A  didt=-750 A/us  trr_factor=3  trr=115 ns  Qrr=150 nA*s  Vr=-600 V  Ls=150 nH  Erec=0.03 J  TT=50 ns  tau=100 ns  T_param=ee.enum.diode.temperatureParam.off  Tdevice=298.15 K  I1_T2=0.245 A  V1_T2=0.5 V  IS_T2=1.25e-7 A  Tmeas2=125 degC  XTI_param=ee.enum.diode.xtiParam.pn  XTI=3  EG_param=ee.enum.diode.egapParam.material_si  EG=1.11 eV  dBVdT=0 V/K  fault_action=simscape.enum.assert.action.none  t_fault=inf s  enable_fault_input=simscape.enum.onoff.off  i_specify=off  i_priority=None  i=0 A  i_nominal_specify=off  i_nominal_value=1  i_nominal_unit=A  v_specify=off  v_priority=None  v=0 V  v_nominal_specify=off  v_nominal_value=1  v_nominal_unit=V  v_capacitor_specify=off  v_capacitor_priority=None  v_capacitor=0 V  v_capacitor_nominal_specify=off  v_capacitor_nominal_value=1  v_capacitor_nominal_unit=V  Qj_specify=off  Qj_priority=High  Qj=0 C  Qj_nominal_specify=off  Qj_nominal_value=1  Qj_nominal_unit=C  i_diode_specify=off  i_diode_priority=None  i_diode=0 A  i_diode_nominal_specify=off  i_diode_nominal_value=1  i_diode_nominal_unit=A  v_diode_specify=off  v_diode_priority=None  v_diode=0 V  v_diode_nominal_specify=off  v_diode_nominal_value=1  v_diode_nominal_unit=V  i_capacitor_specify=off  i_capacitor_priority=None  i_capacitor=0 A  i_capacitor_nominal_specify=off  i_capacitor_nominal_value=1  i_capacitor_nominal_unit=A  power_dissipated_specify=off  power_dissipated_priority=None  power_dissipated=0 W  power_dissipated_nominal_specify=off  power_dissipated_nominal_value=1  power_dissipated_nominal_unit=W  fidelity_level=ee.enum.diode.fidelity.includeChargeDyn  rec_loss_model=ee.enum.diode.reverseRecoveryModel.fixed  ErecVal=0 J  scaleWithIandV=true  ErecMat=zeros(2, 3) J  TjrecVec=[298.15, 398.15] K  IfrecVec=[.1, 1, 10] A  IrecVal=10 A  VrecVal=10 V  tFilter=1 / 1000 / 100 s  thermal_network_parameterization=ee.enum.thermalNetworkTopology.junctionCase  Rth=[0, 10] K/W  Rth_Cauer=[1, 3, 10] K/W  Rth_Foster=[.08, .14, .22, .16] K/W  thermal_mass_parameterization=ee.enum.thermalNetwork.timeconstant  thermal_mass=[0, 1] J/K  thermal_mass_Cauer=[.1, .3, 1] J/K  thermal_mass_Foster=[.001, .005, .05, .5] J/K  thermal_time_constant=[0, 10] s  thermal_time_constant_Cauer=[1, 3, 10] s  thermal_time_constant_Foster=[7e-05, .0007, .01, .08] s  thermal_mass_initial_temperatures=[25, 25] degC  thermal_mass_initial_temperatures_Cauer=[25, 25, 25] degC  junction_thermal_mass=0.01 J/K  Tvec_initial_Foster=[25, 25, 25, 25] degC  no_thermal_network=0  junction_temperature_specify=off  junction_temperature_priority=None  junction_temperature=25 degC  junction_temperature_nominal_specify=off  junction_temperature_nominal_value=1  junction_temperature_nominal_unit=degC
  Phase Splitter : ee_lib/Connectors & References/Phase Splitter
  RCsnuber : Subsystem
  RCsnuber1 : Subsystem
  RCsnuber2 : Subsystem
  RCsnuber3 : Subsystem
  RCsnuber4 : Subsystem
  RCsnuber5 : Subsystem
  abc : PMIOPort  Side=Left
  + : PMIOPort  Port=2  Side=Right
  - : PMIOPort  Port=3  Side=Right
  connections:
  abc/RConn1 -- Phase Splitter/LConn1
  RCsnuber3/RConn1 -- RCsnuber4/RConn1 -- -/RConn1 -- Diode5/LConn1 -- Diode4/LConn1 -- Diode3/LConn1
  RCsnuber2/RConn1 -- Diode1/LConn1 -- Phase Splitter/RConn2 -- RCsnuber4/LConn1 -- Diode4/RConn1
  Diode3/RConn1 -- RCsnuber/RConn1 -- Phase Splitter/RConn1 -- RCsnuber3/LConn1 -- Diode/LConn1
  Diode5/RConn1 -- Diode2/LConn1 -- RCsnuber1/RConn1 -- Phase Splitter/RConn3 -- RCsnuber5/LConn1
  +/RConn1 -- RCsnuber2/LConn1 -- RCsnuber/LConn1 -- Diode2/RConn1 -- Diode1/RConn1 -- Diode/RConn1 -- RCsnuber1/LConn1

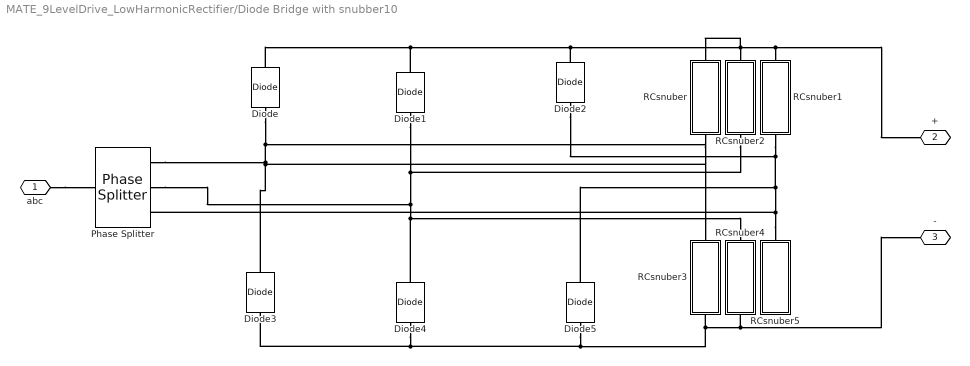
== system MATE_9LevelDrive_LowHarmonicRectifier/Diode Bridge with snubber10 ==
  Diode{,1..5} (6 alike) : ee_lib/Semiconductors & Converters/Diode  ModelType=ee.enum.diode.modelType.pwl  TableType=ee.enum.diode.tableType.IfMat  IfMat=[.07, .12, .19, 1.75, 4.24, 7.32, 11.2; .16, .3, .72, 2.14, 5.02, 8.35, 13.12] A  VfMat=[.9, 1.15, 1.25, 1.5, 1.75, 2.17, 2.6, 2.85; .58, .68, .75, 1.1, 1.38, 1.77, 2.27, 2.7] V  TjVec=[25, 125] degC  VfVec=[.5, .7, .9, 1.3, 1.7, 2.1, 2.5] V  IfVec=[.1, .2, .5, 1, 2, 4, 7, 10] A  IrMat=[1e-06, 2e-06, 5e-06, 1e-05, 2.5e-05, 5e-05, .0001; 2e-06, 5e-06, 1e-05, 4e-05, 8e-05, .0002, .0005] A  VrMat=[10, 100, 200, 250, 300, 325, 350; 10, 70, 160, 220, 270, 300, 320] V  VrVec=[10, 20, 40, 50, 70, 80, 100] V  IrVec=[1e-06, 2e-06, 5e-06, 1e-05, 2e-05, 5e-05, .0001] A  Vf=1 V  Ron=0.01 Ohm  Goff=1e-8 S  prmExp=ee.enum.diode.expParam.useTwo  I12=[.0137, .545] A  V12=[.6, .7] V  RS=0 Ohm  Tmeas=298.15 K  IS=1e-12 A  ec=1  I1=0.0137 A  V1=0.6 V  N_series=1  N_parallel=1  ZenerEnable=false  Rz=0.3 Ohm  BV=inf V  C_param=ee.enum.diode.capParam.fixed  CJ=0 pF  CJ0=5 pF  Vvec=[.1, 10, 100] V  Cvec=[3.5, 1, .4] pF  VJ=1 V  Mgrad=0.5  FC=0.5  Q_param=ee.enum.diode.recoveryParam.off  iRM=-7.15 A  iF=4 A  didt=-750 A/us  trr_factor=3  trr=115 ns  Qrr=150 nA*s  Vr=-600 V  Ls=150 nH  Erec=0.03 J  TT=50 ns  tau=100 ns  T_param=ee.enum.diode.temperatureParam.off  Tdevice=298.15 K  I1_T2=0.245 A  V1_T2=0.5 V  IS_T2=1.25e-7 A  Tmeas2=125 degC  XTI_param=ee.enum.diode.xtiParam.pn  XTI=3  EG_param=ee.enum.diode.egapParam.material_si  EG=1.11 eV  dBVdT=0 V/K  fault_action=simscape.enum.assert.action.none  t_fault=inf s  enable_fault_input=simscape.enum.onoff.off  i_specify=off  i_priority=None  i=0 A  i_nominal_specify=off  i_nominal_value=1  i_nominal_unit=A  v_specify=off  v_priority=None  v=0 V  v_nominal_specify=off  v_nominal_value=1  v_nominal_unit=V  v_capacitor_specify=off  v_capacitor_priority=None  v_capacitor=0 V  v_capacitor_nominal_specify=off  v_capacitor_nominal_value=1  v_capacitor_nominal_unit=V  Qj_specify=off  Qj_priority=High  Qj=0 C  Qj_nominal_specify=off  Qj_nominal_value=1  Qj_nominal_unit=C  i_diode_specify=off  i_diode_priority=None  i_diode=0 A  i_diode_nominal_specify=off  i_diode_nominal_value=1  i_diode_nominal_unit=A  v_diode_specify=off  v_diode_priority=None  v_diode=0 V  v_diode_nominal_specify=off  v_diode_nominal_value=1  v_diode_nominal_unit=V  i_capacitor_specify=off  i_capacitor_priority=None  i_capacitor=0 A  i_capacitor_nominal_specify=off  i_capacitor_nominal_value=1  i_capacitor_nominal_unit=A  power_dissipated_specify=off  power_dissipated_priority=None  power_dissipated=0 W  power_dissipated_nominal_specify=off  power_dissipated_nominal_value=1  power_dissipated_nominal_unit=W  fidelity_level=ee.enum.diode.fidelity.includeChargeDyn  rec_loss_model=ee.enum.diode.reverseRecoveryModel.fixed  ErecVal=0 J  scaleWithIandV=true  ErecMat=zeros(2, 3) J  TjrecVec=[298.15, 398.15] K  IfrecVec=[.1, 1, 10] A  IrecVal=10 A  VrecVal=10 V  tFilter=1 / 1000 / 100 s  thermal_network_parameterization=ee.enum.thermalNetworkTopology.junctionCase  Rth=[0, 10] K/W  Rth_Cauer=[1, 3, 10] K/W  Rth_Foster=[.08, .14, .22, .16] K/W  thermal_mass_parameterization=ee.enum.thermalNetwork.timeconstant  thermal_mass=[0, 1] J/K  thermal_mass_Cauer=[.1, .3, 1] J/K  thermal_mass_Foster=[.001, .005, .05, .5] J/K  thermal_time_constant=[0, 10] s  thermal_time_constant_Cauer=[1, 3, 10] s  thermal_time_constant_Foster=[7e-05, .0007, .01, .08] s  thermal_mass_initial_temperatures=[25, 25] degC  thermal_mass_initial_temperatures_Cauer=[25, 25, 25] degC  junction_thermal_mass=0.01 J/K  Tvec_initial_Foster=[25, 25, 25, 25] degC  no_thermal_network=0  junction_temperature_specify=off  junction_temperature_priority=None  junction_temperature=25 degC  junction_temperature_nominal_specify=off  junction_temperature_nominal_value=1  junction_temperature_nominal_unit=degC
  Phase Splitter : ee_lib/Connectors & References/Phase Splitter
  RCsnuber : Subsystem
  RCsnuber1 : Subsystem
  RCsnuber2 : Subsystem
  RCsnuber3 : Subsystem
  RCsnuber4 : Subsystem
  RCsnuber5 : Subsystem
  abc : PMIOPort  Side=Left
  + : PMIOPort  Port=2  Side=Right
  - : PMIOPort  Port=3  Side=Right
  connections:
  RCsnuber1/LConn1 -- Diode/RConn1 -- Diode1/RConn1 -- Diode2/RConn1 -- RCsnuber/LConn1 -- RCsnuber2/LConn1 -- +/RConn1
  RCsnuber5/LConn1 -- Phase Splitter/RConn3 -- RCsnuber1/RConn1 -- Diode2/LConn1 -- Diode5/RConn1
  Diode/LConn1 -- RCsnuber3/LConn1 -- Phase Splitter/RConn1 -- RCsnuber/RConn1 -- Diode3/RConn1
  Diode4/RConn1 -- RCsnuber4/LConn1 -- Phase Splitter/RConn2 -- Diode1/LConn1 -- RCsnuber2/RConn1
  Diode3/LConn1 -- Diode4/LConn1 -- Diode5/LConn1 -- -/RConn1 -- RCsnuber4/RConn1 -- RCsnuber3/RConn1
  abc/RConn1 -- Phase Splitter/LConn1

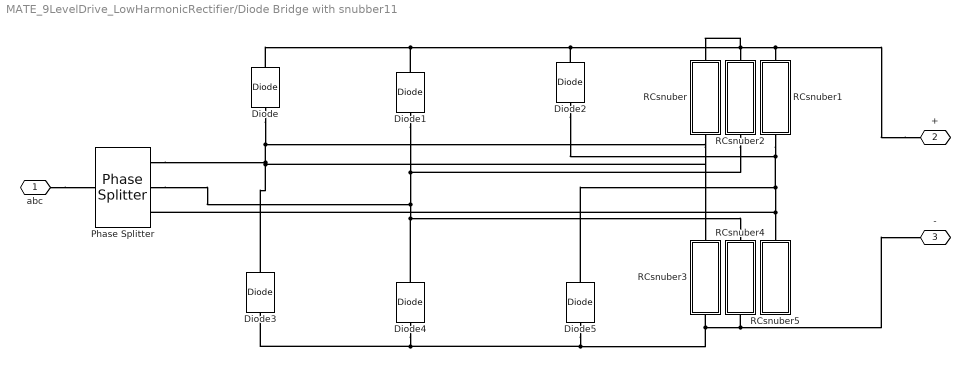
== system MATE_9LevelDrive_LowHarmonicRectifier/Diode Bridge with snubber11 ==
  Diode{,1..5} (6 alike) : ee_lib/Semiconductors & Converters/Diode  ModelType=ee.enum.diode.modelType.pwl  TableType=ee.enum.diode.tableType.IfMat  IfMat=[.07, .12, .19, 1.75, 4.24, 7.32, 11.2; .16, .3, .72, 2.14, 5.02, 8.35, 13.12] A  VfMat=[.9, 1.15, 1.25, 1.5, 1.75, 2.17, 2.6, 2.85; .58, .68, .75, 1.1, 1.38, 1.77, 2.27, 2.7] V  TjVec=[25, 125] degC  VfVec=[.5, .7, .9, 1.3, 1.7, 2.1, 2.5] V  IfVec=[.1, .2, .5, 1, 2, 4, 7, 10] A  IrMat=[1e-06, 2e-06, 5e-06, 1e-05, 2.5e-05, 5e-05, .0001; 2e-06, 5e-06, 1e-05, 4e-05, 8e-05, .0002, .0005] A  VrMat=[10, 100, 200, 250, 300, 325, 350; 10, 70, 160, 220, 270, 300, 320] V  VrVec=[10, 20, 40, 50, 70, 80, 100] V  IrVec=[1e-06, 2e-06, 5e-06, 1e-05, 2e-05, 5e-05, .0001] A  Vf=1 V  Ron=0.01 Ohm  Goff=1e-8 S  prmExp=ee.enum.diode.expParam.useTwo  I12=[.0137, .545] A  V12=[.6, .7] V  RS=0 Ohm  Tmeas=298.15 K  IS=1e-12 A  ec=1  I1=0.0137 A  V1=0.6 V  N_series=1  N_parallel=1  ZenerEnable=false  Rz=0.3 Ohm  BV=inf V  C_param=ee.enum.diode.capParam.fixed  CJ=0 pF  CJ0=5 pF  Vvec=[.1, 10, 100] V  Cvec=[3.5, 1, .4] pF  VJ=1 V  Mgrad=0.5  FC=0.5  Q_param=ee.enum.diode.recoveryParam.off  iRM=-7.15 A  iF=4 A  didt=-750 A/us  trr_factor=3  trr=115 ns  Qrr=150 nA*s  Vr=-600 V  Ls=150 nH  Erec=0.03 J  TT=50 ns  tau=100 ns  T_param=ee.enum.diode.temperatureParam.off  Tdevice=298.15 K  I1_T2=0.245 A  V1_T2=0.5 V  IS_T2=1.25e-7 A  Tmeas2=125 degC  XTI_param=ee.enum.diode.xtiParam.pn  XTI=3  EG_param=ee.enum.diode.egapParam.material_si  EG=1.11 eV  dBVdT=0 V/K  fault_action=simscape.enum.assert.action.none  t_fault=inf s  enable_fault_input=simscape.enum.onoff.off  i_specify=off  i_priority=None  i=0 A  i_nominal_specify=off  i_nominal_value=1  i_nominal_unit=A  v_specify=off  v_priority=None  v=0 V  v_nominal_specify=off  v_nominal_value=1  v_nominal_unit=V  v_capacitor_specify=off  v_capacitor_priority=None  v_capacitor=0 V  v_capacitor_nominal_specify=off  v_capacitor_nominal_value=1  v_capacitor_nominal_unit=V  Qj_specify=off  Qj_priority=High  Qj=0 C  Qj_nominal_specify=off  Qj_nominal_value=1  Qj_nominal_unit=C  i_diode_specify=off  i_diode_priority=None  i_diode=0 A  i_diode_nominal_specify=off  i_diode_nominal_value=1  i_diode_nominal_unit=A  v_diode_specify=off  v_diode_priority=None  v_diode=0 V  v_diode_nominal_specify=off  v_diode_nominal_value=1  v_diode_nominal_unit=V  i_capacitor_specify=off  i_capacitor_priority=None  i_capacitor=0 A  i_capacitor_nominal_specify=off  i_capacitor_nominal_value=1  i_capacitor_nominal_unit=A  power_dissipated_specify=off  power_dissipated_priority=None  power_dissipated=0 W  power_dissipated_nominal_specify=off  power_dissipated_nominal_value=1  power_dissipated_nominal_unit=W  fidelity_level=ee.enum.diode.fidelity.includeChargeDyn  rec_loss_model=ee.enum.diode.reverseRecoveryModel.fixed  ErecVal=0 J  scaleWithIandV=true  ErecMat=zeros(2, 3) J  TjrecVec=[298.15, 398.15] K  IfrecVec=[.1, 1, 10] A  IrecVal=10 A  VrecVal=10 V  tFilter=1 / 1000 / 100 s  thermal_network_parameterization=ee.enum.thermalNetworkTopology.junctionCase  Rth=[0, 10] K/W  Rth_Cauer=[1, 3, 10] K/W  Rth_Foster=[.08, .14, .22, .16] K/W  thermal_mass_parameterization=ee.enum.thermalNetwork.timeconstant  thermal_mass=[0, 1] J/K  thermal_mass_Cauer=[.1, .3, 1] J/K  thermal_mass_Foster=[.001, .005, .05, .5] J/K  thermal_time_constant=[0, 10] s  thermal_time_constant_Cauer=[1, 3, 10] s  thermal_time_constant_Foster=[7e-05, .0007, .01, .08] s  thermal_mass_initial_temperatures=[25, 25] degC  thermal_mass_initial_temperatures_Cauer=[25, 25, 25] degC  junction_thermal_mass=0.01 J/K  Tvec_initial_Foster=[25, 25, 25, 25] degC  no_thermal_network=0  junction_temperature_specify=off  junction_temperature_priority=None  junction_temperature=25 degC  junction_temperature_nominal_specify=off  junction_temperature_nominal_value=1  junction_temperature_nominal_unit=degC
  Phase Splitter : ee_lib/Connectors & References/Phase Splitter
  RCsnuber : Subsystem
  RCsnuber1 : Subsystem
  RCsnuber2 : Subsystem
  RCsnuber3 : Subsystem
  RCsnuber4 : Subsystem
  RCsnuber5 : Subsystem
  abc : PMIOPort  Side=Left
  + : PMIOPort  Port=2  Side=Right
  - : PMIOPort  Port=3  Side=Right
  connections:
  abc/RConn1 -- Phase Splitter/LConn1
  RCsnuber3/RConn1 -- RCsnuber4/RConn1 -- -/RConn1 -- Diode5/LConn1 -- Diode4/LConn1 -- Diode3/LConn1
  RCsnuber2/RConn1 -- Diode1/LConn1 -- Phase Splitter/RConn2 -- RCsnuber4/LConn1 -- Diode4/RConn1
  Diode3/RConn1 -- RCsnuber/RConn1 -- Phase Splitter/RConn1 -- RCsnuber3/LConn1 -- Diode/LConn1
  Diode5/RConn1 -- Diode2/LConn1 -- RCsnuber1/RConn1 -- Phase Splitter/RConn3 -- RCsnuber5/LConn1
  +/RConn1 -- RCsnuber2/LConn1 -- RCsnuber/LConn1 -- Diode2/RConn1 -- Diode1/RConn1 -- Diode/RConn1 -- RCsnuber1/LConn1

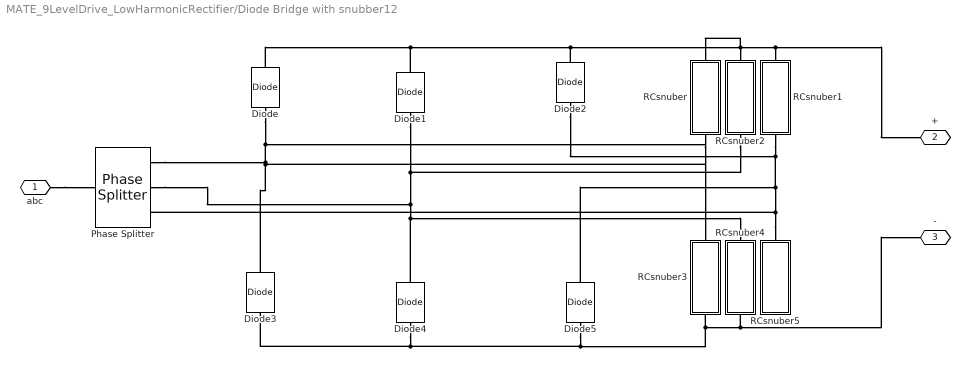
== system MATE_9LevelDrive_LowHarmonicRectifier/Diode Bridge with snubber12 ==
  Diode{,1..5} (6 alike) : ee_lib/Semiconductors & Converters/Diode  ModelType=ee.enum.diode.modelType.pwl  TableType=ee.enum.diode.tableType.IfMat  IfMat=[.07, .12, .19, 1.75, 4.24, 7.32, 11.2; .16, .3, .72, 2.14, 5.02, 8.35, 13.12] A  VfMat=[.9, 1.15, 1.25, 1.5, 1.75, 2.17, 2.6, 2.85; .58, .68, .75, 1.1, 1.38, 1.77, 2.27, 2.7] V  TjVec=[25, 125] degC  VfVec=[.5, .7, .9, 1.3, 1.7, 2.1, 2.5] V  IfVec=[.1, .2, .5, 1, 2, 4, 7, 10] A  IrMat=[1e-06, 2e-06, 5e-06, 1e-05, 2.5e-05, 5e-05, .0001; 2e-06, 5e-06, 1e-05, 4e-05, 8e-05, .0002, .0005] A  VrMat=[10, 100, 200, 250, 300, 325, 350; 10, 70, 160, 220, 270, 300, 320] V  VrVec=[10, 20, 40, 50, 70, 80, 100] V  IrVec=[1e-06, 2e-06, 5e-06, 1e-05, 2e-05, 5e-05, .0001] A  Vf=1 V  Ron=0.01 Ohm  Goff=1e-8 S  prmExp=ee.enum.diode.expParam.useTwo  I12=[.0137, .545] A  V12=[.6, .7] V  RS=0 Ohm  Tmeas=298.15 K  IS=1e-12 A  ec=1  I1=0.0137 A  V1=0.6 V  N_series=1  N_parallel=1  ZenerEnable=false  Rz=0.3 Ohm  BV=inf V  C_param=ee.enum.diode.capParam.fixed  CJ=0 pF  CJ0=5 pF  Vvec=[.1, 10, 100] V  Cvec=[3.5, 1, .4] pF  VJ=1 V  Mgrad=0.5  FC=0.5  Q_param=ee.enum.diode.recoveryParam.off  iRM=-7.15 A  iF=4 A  didt=-750 A/us  trr_factor=3  trr=115 ns  Qrr=150 nA*s  Vr=-600 V  Ls=150 nH  Erec=0.03 J  TT=50 ns  tau=100 ns  T_param=ee.enum.diode.temperatureParam.off  Tdevice=298.15 K  I1_T2=0.245 A  V1_T2=0.5 V  IS_T2=1.25e-7 A  Tmeas2=125 degC  XTI_param=ee.enum.diode.xtiParam.pn  XTI=3  EG_param=ee.enum.diode.egapParam.material_si  EG=1.11 eV  dBVdT=0 V/K  fault_action=simscape.enum.assert.action.none  t_fault=inf s  enable_fault_input=simscape.enum.onoff.off  i_specify=off  i_priority=None  i=0 A  i_nominal_specify=off  i_nominal_value=1  i_nominal_unit=A  v_specify=off  v_priority=None  v=0 V  v_nominal_specify=off  v_nominal_value=1  v_nominal_unit=V  v_capacitor_specify=off  v_capacitor_priority=None  v_capacitor=0 V  v_capacitor_nominal_specify=off  v_capacitor_nominal_value=1  v_capacitor_nominal_unit=V  Qj_specify=off  Qj_priority=High  Qj=0 C  Qj_nominal_specify=off  Qj_nominal_value=1  Qj_nominal_unit=C  i_diode_specify=off  i_diode_priority=None  i_diode=0 A  i_diode_nominal_specify=off  i_diode_nominal_value=1  i_diode_nominal_unit=A  v_diode_specify=off  v_diode_priority=None  v_diode=0 V  v_diode_nominal_specify=off  v_diode_nominal_value=1  v_diode_nominal_unit=V  i_capacitor_specify=off  i_capacitor_priority=None  i_capacitor=0 A  i_capacitor_nominal_specify=off  i_capacitor_nominal_value=1  i_capacitor_nominal_unit=A  power_dissipated_specify=off  power_dissipated_priority=None  power_dissipated=0 W  power_dissipated_nominal_specify=off  power_dissipated_nominal_value=1  power_dissipated_nominal_unit=W  fidelity_level=ee.enum.diode.fidelity.includeChargeDyn  rec_loss_model=ee.enum.diode.reverseRecoveryModel.fixed  ErecVal=0 J  scaleWithIandV=true  ErecMat=zeros(2, 3) J  TjrecVec=[298.15, 398.15] K  IfrecVec=[.1, 1, 10] A  IrecVal=10 A  VrecVal=10 V  tFilter=1 / 1000 / 100 s  thermal_network_parameterization=ee.enum.thermalNetworkTopology.junctionCase  Rth=[0, 10] K/W  Rth_Cauer=[1, 3, 10] K/W  Rth_Foster=[.08, .14, .22, .16] K/W  thermal_mass_parameterization=ee.enum.thermalNetwork.timeconstant  thermal_mass=[0, 1] J/K  thermal_mass_Cauer=[.1, .3, 1] J/K  thermal_mass_Foster=[.001, .005, .05, .5] J/K  thermal_time_constant=[0, 10] s  thermal_time_constant_Cauer=[1, 3, 10] s  thermal_time_constant_Foster=[7e-05, .0007, .01, .08] s  thermal_mass_initial_temperatures=[25, 25] degC  thermal_mass_initial_temperatures_Cauer=[25, 25, 25] degC  junction_thermal_mass=0.01 J/K  Tvec_initial_Foster=[25, 25, 25, 25] degC  no_thermal_network=0  junction_temperature_specify=off  junction_temperature_priority=None  junction_temperature=25 degC  junction_temperature_nominal_specify=off  junction_temperature_nominal_value=1  junction_temperature_nominal_unit=degC
  Phase Splitter : ee_lib/Connectors & References/Phase Splitter
  RCsnuber : Subsystem
  RCsnuber1 : Subsystem
  RCsnuber2 : Subsystem
  RCsnuber3 : Subsystem
  RCsnuber4 : Subsystem
  RCsnuber5 : Subsystem
  abc : PMIOPort  Side=Left
  + : PMIOPort  Port=2  Side=Right
  - : PMIOPort  Port=3  Side=Right
  connections:
  RCsnuber1/LConn1 -- Diode/RConn1 -- Diode1/RConn1 -- Diode2/RConn1 -- RCsnuber/LConn1 -- RCsnuber2/LConn1 -- +/RConn1
  RCsnuber5/LConn1 -- Phase Splitter/RConn3 -- RCsnuber1/RConn1 -- Diode2/LConn1 -- Diode5/RConn1
  Diode/LConn1 -- RCsnuber3/LConn1 -- Phase Splitter/RConn1 -- RCsnuber/RConn1 -- Diode3/RConn1
  Diode4/RConn1 -- RCsnuber4/LConn1 -- Phase Splitter/RConn2 -- Diode1/LConn1 -- RCsnuber2/RConn1
  Diode3/LConn1 -- Diode4/LConn1 -- Diode5/LConn1 -- -/RConn1 -- RCsnuber4/RConn1 -- RCsnuber3/RConn1
  abc/RConn1 -- Phase Splitter/LConn1
